simulink model "BaseEngineController_LS_112"  (Simulink 7.7)
settings: Solver=FixedStepDiscrete  StartTime=0.0  StopTime=10.0  RelTol=1e-3
PreLoadFcn:
  | try, eval([bdroot '_setup']); catch, eval('model_setup', ''); end
InitFcn:
  | try, eval([bdroot '_setup']); catch, eval('model_setup', ''); end
undefined symbols (not defined in the file): ECM, H1, H2, High, motohawk_build_version, motohawk_trunc_name, motohawk_vardec_config_group, motohawk_vardec_path, True, xD
libraries: MotoHawk_lib x1417, motohawk_control_primitives_lib x183, motohawk_engine_lib x32, simulink x21, motohawk_annotations_lib x9, AutoDoc_lib x8, simulink_extras x4, motohawk_ccp_examples_lib x1, motohawk_control_primitives_motoshare_lib x1
(part 24 of 27)

== system BaseEngineController_LS_112/Foreground/Control/VirtualSensors/RawProcessed/Base TPS Request/Variable Rate Limiter ==
  note: Rate Limiter - Limit allowable change in signal per timestep
  input : Inport
  rise rate : Inport  Port=2
  fall rate : Inport  Port=3
  Product : Product  SaturateOnIntegerOverflow=on  InputSameDT=on  OutDataTypeStr=Inherit: Same as first input
  Product1 : Product  Inputs=/*  SaturateOnIntegerOverflow=on  InputSameDT=on  OutDataTypeStr=Inherit: Same as first input
  Saturation : motohawk_control_primitives_lib/Saturation  SystemSampleTime=-1
  Sum2 : Sum  Inputs=|++  SaturateOnIntegerOverflow=on  InputSameDT=on  OutDataTypeStr=Inherit: Same as first input
  Sum3 : Sum  Inputs=|+-  SaturateOnIntegerOverflow=on  InputSameDT=on  OutDataTypeStr=Inherit: Same as first input
  Unit Delay : UnitDelay  SampleTime=-1
  motohawk_delta_time : MotoHawk_lib/Extra Development Blocks/motohawk_delta_time  samp_time=-1  init_val=.005  mode=Seconds (double)
  output : Outport  InitialOutput=0
  wires:
  motohawk_delta_time/1 -> Product/1, Product1/1
  Sum3/1 -> Product1/2
  rise rate/1 -> Saturation/3  "Hi Lim"
  fall rate/1 -> Saturation/2  "Lo Lim"
  Product/1 -> Sum2/1
  Sum2/1 -> output/1, Unit Delay/1
  Unit Delay/1 -> Sum2/2, Sum3/2
  Product1/1 -> Saturation/1  "Slope"
  input/1 -> Sum3/1
  Saturation/1 -> Product/2

== system BaseEngineController_LS_112/Foreground/Control/VirtualSensors/RawProcessed/Capture ECT At Startup/Collect Average ==
  note: Collect samples by summing,
      | and divide by the total, to obtain average
  Count : Inport
  Signal : Inport  Port=2
  Enable : EnablePort  StatesWhenEnabling=reset
  Data Type Conversion : DataTypeConversion  SaturateOnIntegerOverflow=on  RndMeth=Zero
  Product : Product  Inputs=/*  OutDataTypeStr=Inherit: Same as first input
  Sum1 : Sum  Inputs=|++  InputSameDT=on
  Unit Delay1 : UnitDelay  SampleTime=-1
  Captured_Signal : Outport
  wires:
  Unit Delay1/1 -> Sum1/2
  Sum1/1 -> Unit Delay1/1, Product/2
  Signal/1 -> Sum1/1
  Product/1 -> Captured_Signal/1
  Count/1 -> Data Type Conversion/1
  Data Type Conversion/1 -> Product/1

== system BaseEngineController_LS_112/Foreground/Control/VirtualSensors/RawProcessed/Capture IAT At Startup/Collect Average ==
  note: Collect samples by summing,
      | and divide by the total, to obtain average
  Count : Inport
  Signal : Inport  Port=2
  Enable : EnablePort  StatesWhenEnabling=reset
  Data Type Conversion : DataTypeConversion  SaturateOnIntegerOverflow=on  RndMeth=Zero
  Product : Product  Inputs=/*  OutDataTypeStr=Inherit: Same as first input
  Sum1 : Sum  Inputs=|++  InputSameDT=on
  Unit Delay1 : UnitDelay  SampleTime=-1
  Captured_Signal : Outport
  wires:
  Data Type Conversion/1 -> Product/1
  Count/1 -> Data Type Conversion/1
  Product/1 -> Captured_Signal/1
  Signal/1 -> Sum1/1
  Sum1/1 -> Product/2, Unit Delay1/1
  Unit Delay1/1 -> Sum1/2

== system BaseEngineController_LS_112/Foreground/Control/VirtualSensors/RawProcessed/EngineState/TDC_Counter ==
  State : Inport
  f : TriggerPort  TriggerType=function-call
  Constant : Constant  OutDataTypeStr=uint8
  Constant1 : Constant  Value=0  OutDataTypeStr=uint8
  Crank State : motohawk_control_primitives_lib/CompareTo  SystemSampleTime=-1  op===  val=2
  CrankCounter : UnitDelay  SampleTime=-1
  Sum : Sum  Inputs=++|  SaturateOnIntegerOverflow=on
  Switch : Switch  Threshold=1  ZeroCross=off  SaturateOnIntegerOverflow=on  InputSameDT=on
  motohawk_probe1 : MotoHawk_lib/Calibration & Probing Blocks/motohawk_probe  nam='CrankTDCs'  show_more=on  name_source=Use Parameter  read_level=1  view_as=Number  enum_struct={'Disabled', 'Enabled'}  vector_style=Wide Row  use_help_units=off  help=''  units=''  use_header_enum=off  row_header_enum={}  col_header_enum={}  use_precision=off  precision=''  gain=1  offset=0  exp=1  use_mototune_group=on  mototune_group=motohawk_vardec_path(gcb)
  CrankCount : Outport
  wires:
  Constant1/1 -> Switch/3
  Sum/1 -> Switch/1
  Switch/1 -> motohawk_probe1/1, CrankCount/1, CrankCounter/1
  Crank State/1 -> Switch/2
  CrankCounter/1 -> Sum/1
  Constant/1 -> Sum/2
  State/1 -> Crank State/1

== system BaseEngineController_LS_112/Foreground/Inputs/LinearSensors/FuelOxygenationSensor/Filter Options/Moving Average Filter ==
  In1 : Inport
  Product{,1..3} (4 alike) : Product  RndMeth=Zero
  Sum : Sum
  Sum1 : Sum  Inputs=++|
  Sum2 : Sum  Inputs=++|
  Unit Delay : UnitDelay  SampleTime=-1
  Unit Delay1 : UnitDelay  SampleTime=-1
  Unit Delay2 : UnitDelay  SampleTime=-1
  motohawk_calibration : MotoHawk_lib/Calibration & Probing Blocks/motohawk_calibration  nam='FinalGain'  val=.5  storage=Calibration  show_more=on  name_source=Use Parameter  data_type=Inherit from 'Default Value'  read_level=1  write_level=1  ovr_cals=on  view_as=Number  enum_struct={'Disabled', 'Enabled'}  vector_style=Wide Row  use_help_units=on  help='Gain 4 For Moving Average Filter'  units=''  use_header_enum=off  row_header_enum={}  col_header_enum={}  use_min_max=off  min_val=-inf  max_val=inf  use_precision=off  precision=''  gain=1  offset=0  exp=1  use_mototune_group=off  mototune_group=motohawk_vardec_path(gcb)
  motohawk_calibration1 : MotoHawk_lib/Calibration & Probing Blocks/motohawk_calibration  nam='Gain1'  val=.5  storage=Calibration  show_more=on  name_source=Use Parameter  data_type=Inherit from 'Default Value'  read_level=1  write_level=1  ovr_cals=on  view_as=Number  enum_struct={'Disabled', 'Enabled'}  vector_style=Wide Row  use_help_units=on  help='Gain 1 For Moving Average Filter'  units=''  use_header_enum=off  row_header_enum={}  col_header_enum={}  use_min_max=off  min_val=-inf  max_val=inf  use_precision=off  precision=''  gain=1  offset=0  exp=1  use_mototune_group=off  mototune_group=motohawk_vardec_path(gcb)
  motohawk_calibration2 : MotoHawk_lib/Calibration & Probing Blocks/motohawk_calibration  nam='Gain2'  val=.3  storage=Calibration  show_more=on  name_source=Use Parameter  data_type=Inherit from 'Default Value'  read_level=1  write_level=1  ovr_cals=on  view_as=Number  enum_struct={'Disabled', 'Enabled'}  vector_style=Wide Row  use_help_units=on  help='Gain 2 For Moving Average Filter'  units=''  use_header_enum=off  row_header_enum={}  col_header_enum={}  use_min_max=off  min_val=-inf  max_val=inf  use_precision=off  precision=''  gain=1  offset=0  exp=1  use_mototune_group=off  mototune_group=motohawk_vardec_path(gcb)
  motohawk_calibration3 : MotoHawk_lib/Calibration & Probing Blocks/motohawk_calibration  nam='Gain3'  val=.2  storage=Calibration  show_more=on  name_source=Use Parameter  data_type=Inherit from 'Default Value'  read_level=1  write_level=1  ovr_cals=on  view_as=Number  enum_struct={'Disabled', 'Enabled'}  vector_style=Wide Row  use_help_units=on  help='Gain 3 For Moving Average Filter'  units=''  use_header_enum=off  row_header_enum={}  col_header_enum={}  use_min_max=off  min_val=-inf  max_val=inf  use_precision=off  precision=''  gain=1  offset=0  exp=1  use_mototune_group=off  mototune_group=motohawk_vardec_path(gcb)
  Out1 : Outport
  wires:
  Sum/1 -> Product/2
  Product/1 -> Out1/1
  motohawk_calibration/1 -> Product/1
  In1/1 -> Sum/1, Unit Delay/1
  Unit Delay/1 -> Unit Delay1/1, Product1/2
  Unit Delay1/1 -> Unit Delay2/1, Product2/2
  Unit Delay2/1 -> Product3/2
  motohawk_calibration1/1 -> Product1/1
  motohawk_calibration3/1 -> Product3/1
  motohawk_calibration2/1 -> Product2/1
  Product1/1 -> Sum1/1
  Product2/1 -> Sum2/1
  Sum2/1 -> Sum1/2
  Sum1/1 -> Sum/2
  Product3/1 -> Sum2/2

== system BaseEngineController_LS_112/Foreground/Inputs/LinearSensors/FuelOxygenationSensor/Filter Options/Rate Limiter ==
  In1 : Inport
  Variable Rate Limiter : motohawk_control_primitives_motoshare_lib/Variable Rate Limiter  SystemSampleTime=-1
  motohawk_calibration : MotoHawk_lib/Calibration & Probing Blocks/motohawk_calibration  nam='Rise_Rate'  val=.025  storage=Calibration  show_more=off  name_source=Use Parameter  data_type=Inherit from 'Default Value'  read_level=1  write_level=1  ovr_cals=on  view_as=Number  enum_struct={'Disabled', 'Enabled'}  vector_style=Wide Row  use_help_units=off  help=''  units=''  use_header_enum=off  row_header_enum={}  col_header_enum={}  use_min_max=off  min_val=-inf  max_val=inf  use_precision=off  precision=''  gain=1  offset=0  exp=1  use_mototune_group=off  mototune_group=motohawk_vardec_path(gcb)
  motohawk_calibration1 : MotoHawk_lib/Calibration & Probing Blocks/motohawk_calibration  nam='Fall_Rate'  val=.025  storage=Calibration  show_more=off  name_source=Use Parameter  data_type=Inherit from 'Default Value'  read_level=1  write_level=1  ovr_cals=on  view_as=Number  enum_struct={'Disabled', 'Enabled'}  vector_style=Wide Row  use_help_units=off  help=''  units=''  use_header_enum=off  row_header_enum={}  col_header_enum={}  use_min_max=off  min_val=-inf  max_val=inf  use_precision=off  precision=''  gain=1  offset=0  exp=1  use_mototune_group=off  mototune_group=motohawk_vardec_path(gcb)
  Out1 : Outport
  wires:
  Variable Rate Limiter/1 -> Out1/1
  In1/1 -> Variable Rate Limiter/1
  motohawk_calibration/1 -> Variable Rate Limiter/2
  motohawk_calibration1/1 -> Variable Rate Limiter/3

== system BaseEngineController_LS_112/Foreground/Outputs/AEM Infinity Dash/Dash Message 2/PHI_Filt/DecreasingFilter ==
  Enable : EnablePort
  motohawk_calibration2 : MotoHawk_lib/Calibration & Probing Blocks/motohawk_calibration  nam='PH1_FiltDecConst'  val=1.25  storage=Calibration  show_more=on  name_source=Use Parameter  data_type=Inherit from 'Default Value'  read_level=1  write_level=1  ovr_cals=on  view_as=Number  enum_struct={'Disabled', 'Enabled'}  vector_style=Wide Row  use_help_units=on  help='Filter time constant for a decreasing signal.'  units='sec'  use_header_enum=off  row_header_enum={}  col_header_enum={}  use_min_max=off  min_val=-inf  max_val=inf  use_precision=off  precision=''  gain=1  offset=0  exp=1  use_mototune_group=on  mototune_group=motohawk_vardec_path(gcb)
  Out1 : Outport  InitialOutput=.005
  wires:
  motohawk_calibration2/1 -> Out1/1

== system BaseEngineController_LS_112/Foreground/Outputs/AEM Infinity Dash/Dash Message 2/PHI_Filt/IncreasingFilter ==
  Enable : EnablePort
  motohawk_calibration1 : MotoHawk_lib/Calibration & Probing Blocks/motohawk_calibration  nam='PH1_FiltIncConst'  val=1.25  storage=Calibration  show_more=on  name_source=Use Parameter  data_type=Inherit from 'Default Value'  read_level=1  write_level=1  ovr_cals=on  view_as=Number  enum_struct={'Disabled', 'Enabled'}  vector_style=Wide Row  use_help_units=on  help='Filter time constant for a increasing signal.'  units='sec'  use_header_enum=off  row_header_enum={}  col_header_enum={}  use_min_max=off  min_val=-inf  max_val=inf  use_precision=off  precision=''  gain=1  offset=0  exp=1  use_mototune_group=on  mototune_group=motohawk_vardec_path(gcb)
  Out1 : Outport  InitialOutput=.005
  wires:
  motohawk_calibration1/1 -> Out1/1

== system BaseEngineController_LS_112/Foreground/Outputs/AEM Infinity Dash/Dash Message 2/PHI_Filt1/DecreasingFilter ==
  Enable : EnablePort
  motohawk_calibration2 : MotoHawk_lib/Calibration & Probing Blocks/motohawk_calibration  nam='PH2_FiltDecConst'  val=1.25  storage=Calibration  show_more=on  name_source=Use Parameter  data_type=Inherit from 'Default Value'  read_level=1  write_level=1  ovr_cals=on  view_as=Number  enum_struct={'Disabled', 'Enabled'}  vector_style=Wide Row  use_help_units=on  help='Filter time constant for a decreasing signal.'  units='sec'  use_header_enum=off  row_header_enum={}  col_header_enum={}  use_min_max=off  min_val=-inf  max_val=inf  use_precision=off  precision=''  gain=1  offset=0  exp=1  use_mototune_group=on  mototune_group=motohawk_vardec_path(gcb)
  Out1 : Outport  InitialOutput=.005
  wires:
  motohawk_calibration2/1 -> Out1/1

== system BaseEngineController_LS_112/Foreground/Outputs/AEM Infinity Dash/Dash Message 2/PHI_Filt1/IncreasingFilter ==
  Enable : EnablePort
  motohawk_calibration1 : MotoHawk_lib/Calibration & Probing Blocks/motohawk_calibration  nam='PH2_FiltIncConst'  val=1.25  storage=Calibration  show_more=on  name_source=Use Parameter  data_type=Inherit from 'Default Value'  read_level=1  write_level=1  ovr_cals=on  view_as=Number  enum_struct={'Disabled', 'Enabled'}  vector_style=Wide Row  use_help_units=on  help='Filter time constant for a increasing signal.'  units='sec'  use_header_enum=off  row_header_enum={}  col_header_enum={}  use_min_max=off  min_val=-inf  max_val=inf  use_precision=off  precision=''  gain=1  offset=0  exp=1  use_mototune_group=on  mototune_group=motohawk_vardec_path(gcb)
  Out1 : Outport  InitialOutput=.005
  wires:
  motohawk_calibration1/1 -> Out1/1

== system BaseEngineController_LS_112/Foreground/Outputs/Coil Control/Coil Enable Manager/EST Enable TDC Counter/TDC_Counter ==
  Reset : Inport
  f : TriggerPort  TriggerType=function-call
  Constant : Constant  OutDataTypeStr=uint8
  Constant1 : Constant  Value=0  OutDataTypeStr=uint8
  CrankCounter : UnitDelay  SampleTime=-1
  Sum : Sum  Inputs=|++  SaturateOnIntegerOverflow=on
  Switch1 : Switch  Threshold=1  ZeroCross=off  SaturateOnIntegerOverflow=on  InputSameDT=on
  CrankCount : Outport
  wires:
  Constant1/1 -> Switch1/1
  Sum/1 -> Switch1/3
  Reset/1 -> Switch1/2
  Switch1/1 -> CrankCount/1, CrankCounter/1
  Constant/1 -> Sum/1
  CrankCounter/1 -> Sum/2

== system BaseEngineController_LS_112/Foreground/Control/ActuatorCharacterization/Electronic Throttle Controller/PID With Damper Terms (Tunable)/DamperSwitch/Filtered Derivative ==
  Raw : Inport
  Derivitive2 : motohawk_control_primitives_lib/Derivitive  SystemSampleTime=-1  samp_time=.005
  First Order Low Pass (Tunable) : motohawk_control_primitives_lib/First Order Low Pass (Tunable)  SystemSampleTime=-1  nam=[prefix 'DamperTPSFilt']  samp_time=-1  group=[grp ' | ' prefix ' PID Config']
  Filt_Deriv : Outport
  wires:
  Raw/1 -> First Order Low Pass (Tunable)/1
  Derivitive2/1 -> Filt_Deriv/1
  First Order Low Pass (Tunable)/1 -> Derivitive2/1

== system BaseEngineController_LS_112/Foreground/Control/Controller/Run/AC Control/AC Comp High Pressure/Hysteresis ==
  note: Hi & !Lo => Hi
      | Lo & !Hi => Lo
      | Otherwise, Hold
  Hi : Inport
  Lo : Inport  Port=2
  Combinatorial  Logic : CombinatorialLogic  TruthTable=[0 0;0 1;1 1;0 0]
  Demux : Demux  Outputs=2
  Mux : Mux  Inputs=2
  Switch1 : Switch  Threshold=0.5  SaturateOnIntegerOverflow=on  InputSameDT=on
  Unit Delay : UnitDelay  SampleTime=-1
  "Out (Lo=0, Hi=1)" : Outport
  wires:
  Mux/1 -> Combinatorial  Logic/1
  Combinatorial  Logic/1 -> Demux/1
  Demux/1 -> Switch1/1
  Demux/2 -> Switch1/2
  Unit Delay/1 -> Switch1/3
  Switch1/1 -> Unit Delay/1, "Out (Lo=0, Hi=1)"/1
  Hi/1 -> Mux/1
  Lo/1 -> Mux/2

== system BaseEngineController_LS_112/Foreground/Control/Controller/Run/AC Control/AC Comp Low Pressure/Hysteresis ==
  note: Hi & !Lo => Hi
      | Lo & !Hi => Lo
      | Otherwise, Hold
  Hi : Inport
  Lo : Inport  Port=2
  Combinatorial  Logic : CombinatorialLogic  TruthTable=[0 0;0 1;1 1;0 0]
  Demux : Demux  Outputs=2
  Mux : Mux  Inputs=2
  Switch1 : Switch  Threshold=0.5  SaturateOnIntegerOverflow=on  InputSameDT=on
  Unit Delay : UnitDelay  SampleTime=-1
  "Out (Lo=0, Hi=1)" : Outport
  wires:
  Mux/1 -> Combinatorial  Logic/1
  Combinatorial  Logic/1 -> Demux/1
  Demux/1 -> Switch1/1
  Demux/2 -> Switch1/2
  Unit Delay/1 -> Switch1/3
  Switch1/1 -> Unit Delay/1, "Out (Lo=0, Hi=1)"/1
  Hi/1 -> Mux/1
  Lo/1 -> Mux/2

== system BaseEngineController_LS_112/Foreground/Control/Controller/Run/AC Control/AC Comp Overspeed/Hysteresis ==
  note: Hi & !Lo => Hi
      | Lo & !Hi => Lo
      | Otherwise, Hold
  Hi : Inport
  Lo : Inport  Port=2
  Combinatorial  Logic : CombinatorialLogic  TruthTable=[0 0;0 1;1 1;0 0]
  Demux : Demux  Outputs=2
  Mux : Mux  Inputs=2
  Switch1 : Switch  Threshold=0.5  SaturateOnIntegerOverflow=on  InputSameDT=on
  Unit Delay : UnitDelay  SampleTime=-1
  "Out (Lo=0, Hi=1)" : Outport
  wires:
  Mux/1 -> Combinatorial  Logic/1
  Combinatorial  Logic/1 -> Demux/1
  Demux/1 -> Switch1/1
  Demux/2 -> Switch1/2
  Unit Delay/1 -> Switch1/3
  Switch1/1 -> Unit Delay/1, "Out (Lo=0, Hi=1)"/1
  Hi/1 -> Mux/1
  Lo/1 -> Mux/2

== system BaseEngineController_LS_112/Foreground/Control/Controller/Run/AC Control/AC Comp Overspeed1/Hysteresis ==
  note: Hi & !Lo => Hi
      | Lo & !Hi => Lo
      | Otherwise, Hold
  Hi : Inport
  Lo : Inport  Port=2
  Combinatorial  Logic : CombinatorialLogic  TruthTable=[0 0;0 1;1 1;0 0]
  Demux : Demux  Outputs=2
  Mux : Mux  Inputs=2
  Switch1 : Switch  Threshold=0.5  SaturateOnIntegerOverflow=on  InputSameDT=on
  Unit Delay : UnitDelay  SampleTime=-1
  "Out (Lo=0, Hi=1)" : Outport
  wires:
  Mux/1 -> Combinatorial  Logic/1
  Combinatorial  Logic/1 -> Demux/1
  Demux/1 -> Switch1/1
  Demux/2 -> Switch1/2
  Unit Delay/1 -> Switch1/3
  Switch1/1 -> Unit Delay/1, "Out (Lo=0, Hi=1)"/1
  Hi/1 -> Mux/1
  Lo/1 -> Mux/2

== system BaseEngineController_LS_112/Foreground/Control/Controller/Run/AC Control/AC Comp Underspeed/Hysteresis ==
  note: Hi & !Lo => Hi
      | Lo & !Hi => Lo
      | Otherwise, Hold
  Hi : Inport
  Lo : Inport  Port=2
  Combinatorial  Logic : CombinatorialLogic  TruthTable=[0 0;0 1;1 1;0 0]
  Demux : Demux  Outputs=2
  Mux : Mux  Inputs=2
  Switch1 : Switch  Threshold=0.5  SaturateOnIntegerOverflow=on  InputSameDT=on
  Unit Delay : UnitDelay  SampleTime=-1
  "Out (Lo=0, Hi=1)" : Outport
  wires:
  Mux/1 -> Combinatorial  Logic/1
  Combinatorial  Logic/1 -> Demux/1
  Demux/1 -> Switch1/1
  Demux/2 -> Switch1/2
  Unit Delay/1 -> Switch1/3
  Switch1/1 -> Unit Delay/1, "Out (Lo=0, Hi=1)"/1
  Hi/1 -> Mux/1
  Lo/1 -> Mux/2

== system BaseEngineController_LS_112/Foreground/Control/Controller/Run/AC Control/AC Evap Temp Hyst/Hysteresis ==
  note: Hi & !Lo => Hi
      | Lo & !Hi => Lo
      | Otherwise, Hold
  Hi : Inport
  Lo : Inport  Port=2
  Combinatorial  Logic : CombinatorialLogic  TruthTable=[0 0;0 1;1 1;0 0]
  Demux : Demux  Outputs=2
  Mux : Mux  Inputs=2
  Switch1 : Switch  Threshold=0.5  SaturateOnIntegerOverflow=on  InputSameDT=on
  Unit Delay : UnitDelay  SampleTime=-1
  "Out (Lo=0, Hi=1)" : Outport
  wires:
  Mux/1 -> Combinatorial  Logic/1
  Combinatorial  Logic/1 -> Demux/1
  Demux/1 -> Switch1/1
  Demux/2 -> Switch1/2
  Unit Delay/1 -> Switch1/3
  Switch1/1 -> Unit Delay/1, "Out (Lo=0, Hi=1)"/1
  Hi/1 -> Mux/1
  Lo/1 -> Mux/2

== system BaseEngineController_LS_112/Foreground/Control/Controller/Run/Boost Control/BoostControl Adapt/Adapt Boost Table ==
  error : Inport
  Enable : EnablePort
  Documentation_Calibrations_Probes_Block : AutoDoc_lib/Documentation_Calibrations_Probes_Block
  Documentation_Left_Border : AutoDoc_lib/Documentation_Left_Border  layout=Portrait
  Documentation_Right_Border : AutoDoc_lib/Documentation_Right_Border  layout=Portrait
  motohawk_adapt_table : MotoHawk_lib/Lookup Tables/motohawk_adapt_table  nam='BoostControlBase_AdaptMap'  typ=double  mode=Adapt between points  show_adapted=off
  motohawk_calibration1 : MotoHawk_lib/Calibration & Probing Blocks/motohawk_calibration  nam='BoostControlOfstMinValue'  val=0  storage=Calibration  show_more=on  name_source=Use Parameter  data_type=double  read_level=1  write_level=1  ovr_cals=on  view_as=Number  enum_struct={'Disabled', 'Enabled'}  vector_style=Wide Row  use_help_units=on  help='Minimum value that can be adapted into the BaseAirflowOfst table.'  units='%'  use_header_enum=off  row_header_enum={}  col_header_enum={}  use_min_max=on  min_val=-inf  max_val=inf  use_precision=off  precision=''  gain=1  offset=0  exp=1  use_mototune_group=on  mototune_group=motohawk_vardec_path(gcb)
  motohawk_calibration2 : MotoHawk_lib/Calibration & Probing Blocks/motohawk_calibration  nam='BoostControlOfstMaxValue'  val=0  storage=Calibration  show_more=on  name_source=Use Parameter  data_type=double  read_level=1  write_level=1  ovr_cals=on  view_as=Number  enum_struct={'Disabled', 'Enabled'}  vector_style=Wide Row  use_help_units=on  help='Maximum value that can be adapted into the BaseAirflowOfst table.'  units='%'  use_header_enum=off  row_header_enum={}  col_header_enum={}  use_min_max=on  min_val=-inf  max_val=inf  use_precision=off  precision=''  gain=1  offset=0  exp=1  use_mototune_group=on  mototune_group=motohawk_vardec_path(gcb)
  wires:
  error/1 -> motohawk_adapt_table/1
  motohawk_calibration1/1 -> motohawk_adapt_table/2
  motohawk_calibration2/1 -> motohawk_adapt_table/3

== system BaseEngineController_LS_112/Foreground/Control/Controller/Run/Boost Control/BoostControl Adapt/BoostControl Enable Delay ==
  State_In : Inport
  Relational Operator : RelationalOperator  Operator=>  InputSameDT=on
  Time Since Enabled (With Input)1 : motohawk_control_primitives_lib/Time Since Enabled (With Input)1  SystemSampleTime=-1  nam='BoostTimer'  samp_time=.005  init=0  upperlim=16000
  motohawk_calibration1 : MotoHawk_lib/Calibration & Probing Blocks/motohawk_calibration  nam='BoostAdaptDelayTime'  val=5  storage=Calibration  show_more=on  name_source=Use Parameter  data_type=Inherit from 'Default Value'  read_level=1  write_level=1  ovr_cals=on  view_as=Number  enum_struct={'Disabled', 'Enabled'}  vector_style=Wide Row  use_help_units=on  help='Idle Control must be enabled for this amount of time before fuel adaption is enabled'  units='s'  use_header_enum=off  row_header_enum={}  col_header_enum={}  use_min_max=off  min_val=0  max_val=inf  use_precision=off  precision=''  gain=1  offset=0  exp=1  use_mototune_group=on  mototune_group=motohawk_vardec_path(gcb)
  State_Out : Outport
  wires:
  State_In/1 -> Time Since Enabled (With Input)1/1
  motohawk_calibration1/1 -> Relational Operator/2
  Time Since Enabled (With Input)1/1 -> Relational Operator/1
  Relational Operator/1 -> State_Out/1

== system BaseEngineController_LS_112/Foreground/Control/Controller/Run/Boost Control/BoostControl Adapt/Saturation (Tunable) ==
  note: Calibratable wrapper around the Saturation block
  In : Inport
  Saturation : motohawk_control_primitives_lib/Saturation  SystemSampleTime=-1
  motohawk_calibration : MotoHawk_lib/Calibration & Probing Blocks/motohawk_calibration  nam=[prefix 'LwrLim']  val=LwrLim  storage=Calibration  show_more=on  name_source=Use Parameter  data_type=Inherit via back propagation  read_level=1  write_level=1  ovr_cals=on  view_as=Number  enum_struct={'Disabled', 'Enabled'}  vector_style=Wide Row  use_help_units=off  help='Lower Limit Value'  units=units  use_header_enum=off  row_header_enum={}  col_header_enum={}  use_min_max=on  min_val=-inf  max_val=inf  use_precision=on  precision='1.4'  gain=1  offset=0  exp=1  use_mototune_group=on  mototune_group=motohawk_vardec_path(gcb)
  motohawk_calibration1 : MotoHawk_lib/Calibration & Probing Blocks/motohawk_calibration  nam=[prefix 'UprLim']  val=UprLim  storage=Calibration  show_more=on  name_source=Use Parameter  data_type=Inherit via back propagation  read_level=1  write_level=1  ovr_cals=on  view_as=Number  enum_struct={'Disabled', 'Enabled'}  vector_style=Wide Row  use_help_units=off  help='Upper Limit Value'  units=units  use_header_enum=off  row_header_enum={}  col_header_enum={}  use_min_max=on  min_val=-inf  max_val=inf  use_precision=on  precision='1.4'  gain=1  offset=0  exp=1  use_mototune_group=on  mototune_group=motohawk_vardec_path(gcb)
  Out : Outport
  wires:
  motohawk_calibration1/1 -> Saturation/3
  In/1 -> Saturation/1
  motohawk_calibration/1 -> Saturation/2
  Saturation/1 -> Out/1

== system BaseEngineController_LS_112/Foreground/Control/Controller/Run/Boost Control/Universal PID (Tunable & Scheduled)/PID Gain Select1 ==
  ErrorIdx : Inport
  Product1 : Product  SaturateOnIntegerOverflow=on  InputSameDT=on  OutDataTypeStr=Inherit: Same as first input
  Product2 : Product  SaturateOnIntegerOverflow=on  InputSameDT=on  OutDataTypeStr=Inherit: Same as first input
  Product3 : Product  SaturateOnIntegerOverflow=on  InputSameDT=on  OutDataTypeStr=Inherit: Same as first input
  motohawk_calibration1 : MotoHawk_lib/Calibration & Probing Blocks/motohawk_calibration  nam=[prefix 'IGain']  val=0  storage=Calibration  show_more=on  name_source=Use Parameter  data_type=Inherit from 'Default Value'  read_level=1  write_level=1  ovr_cals=on  view_as=Number  enum_struct={'Disabled', 'Enabled'}  vector_style=Wide Row  use_help_units=on  help='Base I-gain for the min. governor controller.'  units='mult'  use_header_enum=off  row_header_enum={}  col_header_enum={}  use_min_max=off  min_val=-inf  max_val=inf  use_precision=off  precision=''  gain=1  offset=0  exp=1  use_mototune_group=on  mototune_group=motohawk_vardec_path(gcb)
  motohawk_calibration2 : MotoHawk_lib/Calibration & Probing Blocks/motohawk_calibration  nam=[prefix 'DGain']  val=0  storage=Calibration  show_more=on  name_source=Use Parameter  data_type=Inherit from 'Default Value'  read_level=1  write_level=1  ovr_cals=on  view_as=Number  enum_struct={'Disabled', 'Enabled'}  vector_style=Wide Row  use_help_units=on  help='Base D-gain for the min. governor controller.'  units='mult'  use_header_enum=off  row_header_enum={}  col_header_enum={}  use_min_max=off  min_val=-inf  max_val=inf  use_precision=off  precision=''  gain=1  offset=0  exp=1  use_mototune_group=on  mototune_group=motohawk_vardec_path(gcb)
  motohawk_calibration3 : MotoHawk_lib/Calibration & Probing Blocks/motohawk_calibration  nam=[prefix 'PGain']  val=0  storage=Calibration  show_more=on  name_source=Use Parameter  data_type=Inherit from 'Default Value'  read_level=1  write_level=1  ovr_cals=on  view_as=Number  enum_struct={'Disabled', 'Enabled'}  vector_style=Wide Row  use_help_units=on  help='Base P-gain for the min. governor controller.'  units='mult'  use_header_enum=off  row_header_enum={}  col_header_enum={}  use_min_max=off  min_val=-inf  max_val=inf  use_precision=off  precision=''  gain=1  offset=0  exp=1  use_mototune_group=on  mototune_group=motohawk_vardec_path(gcb)
  motohawk_interpolation_1d1 : MotoHawk_lib/Lookup Tables/motohawk_interpolation_1d  nam=[prefix 'IGainErrorMult']  table_data=[0.5 0.3 0.01 0.01 0.2 0.5 1 1.3 1.5]  show_more=on  data_type=Inherit from 'Table Data'  storage=NonAdaptive  read_level=1  write_level=1  ovr_cals=on  use_help=on  help=''  units='mult'  use_min_max=on  min_val=-inf  max_val=inf  use_precision=off  precision=''  gain=1  offset=0  exp=1  use_links=off  prelookup_block=''  output_name=''  use_mototune_group=on  mototune_group=motohawk_vardec_path(gcb)
  motohawk_interpolation_1d2 : MotoHawk_lib/Lookup Tables/motohawk_interpolation_1d  nam=[prefix 'PGainErrorMult']  table_data=[0.5 0.3 0.01 0.01 0.2 0.5 1 1.3 1.5]  show_more=on  data_type=Inherit from 'Table Data'  storage=NonAdaptive  read_level=1  write_level=1  ovr_cals=on  use_help=on  help=''  units='mult'  use_min_max=on  min_val=-inf  max_val=inf  use_precision=off  precision=''  gain=1  offset=0  exp=1  use_links=off  prelookup_block=''  output_name=''  use_mototune_group=on  mototune_group=motohawk_vardec_path(gcb)
  motohawk_interpolation_1d3 : MotoHawk_lib/Lookup Tables/motohawk_interpolation_1d  nam=[prefix 'DGainErrorMult']  table_data=[0.5 0.3 0.01 0.01 0.2 0.5 1 1.3 1.5]  show_more=on  data_type=Inherit from 'Table Data'  storage=NonAdaptive  read_level=1  write_level=1  ovr_cals=on  use_help=on  help=''  units='mult'  use_min_max=on  min_val=-inf  max_val=inf  use_precision=off  precision=''  gain=1  offset=0  exp=1  use_links=off  prelookup_block=''  output_name=''  use_mototune_group=on  mototune_group=motohawk_vardec_path(gcb)
  PGain : Outport
  IGain : Outport  Port=2
  DGain : Outport  Port=3
  wires:
  ErrorIdx/1 -> motohawk_interpolation_1d2/1, motohawk_interpolation_1d1/1, motohawk_interpolation_1d3/1
  motohawk_interpolation_1d2/1 -> Product2/2
  Product2/1 -> PGain/1
  motohawk_calibration3/1 -> Product2/1
  motohawk_calibration1/1 -> Product1/1
  motohawk_interpolation_1d1/1 -> Product1/2
  Product1/1 -> IGain/1
  motohawk_interpolation_1d3/1 -> Product3/2
  Product3/1 -> DGain/1
  motohawk_calibration2/1 -> Product3/1

== system BaseEngineController_LS_112/Foreground/Control/Controller/Run/FAN Control/Hysterisis/Hysteresis ==
  note: Hi & !Lo => Hi
      | Lo & !Hi => Lo
      | Otherwise, Hold
  Hi : Inport
  Lo : Inport  Port=2
  Combinatorial  Logic : CombinatorialLogic  TruthTable=[0 0;0 1;1 1;0 0]
  Demux : Demux  Outputs=2
  Mux : Mux  Inputs=2
  Switch1 : Switch  Threshold=0.5  SaturateOnIntegerOverflow=on  InputSameDT=on
  Unit Delay : UnitDelay  SampleTime=-1
  "Out (Lo=0, Hi=1)" : Outport
  wires:
  Mux/1 -> Combinatorial  Logic/1
  Combinatorial  Logic/1 -> Demux/1
  Demux/1 -> Switch1/1
  Demux/2 -> Switch1/2
  Unit Delay/1 -> Switch1/3
  Switch1/1 -> Unit Delay/1, "Out (Lo=0, Hi=1)"/1
  Hi/1 -> Mux/1
  Lo/1 -> Mux/2

== system BaseEngineController_LS_112/Foreground/Control/Controller/Run/FAN Control/Hysterisis1/Hysteresis ==
  note: Hi & !Lo => Hi
      | Lo & !Hi => Lo
      | Otherwise, Hold
  Hi : Inport
  Lo : Inport  Port=2
  Combinatorial  Logic : CombinatorialLogic  TruthTable=[0 0;0 1;1 1;0 0]
  Demux : Demux  Outputs=2
  Mux : Mux  Inputs=2
  Switch1 : Switch  Threshold=0.5  SaturateOnIntegerOverflow=on  InputSameDT=on
  Unit Delay : UnitDelay  SampleTime=-1
  "Out (Lo=0, Hi=1)" : Outport
  wires:
  Mux/1 -> Combinatorial  Logic/1
  Combinatorial  Logic/1 -> Demux/1
  Demux/1 -> Switch1/1
  Demux/2 -> Switch1/2
  Unit Delay/1 -> Switch1/3
  Switch1/1 -> Unit Delay/1, "Out (Lo=0, Hi=1)"/1
  Hi/1 -> Mux/1
  Lo/1 -> Mux/2

== system BaseEngineController_LS_112/Foreground/Control/Controller/Run/FAN Control/Hysterisis2/Hysteresis ==
  note: Hi & !Lo => Hi
      | Lo & !Hi => Lo
      | Otherwise, Hold
  Hi : Inport
  Lo : Inport  Port=2
  Combinatorial  Logic : CombinatorialLogic  TruthTable=[0 0;0 1;1 1;0 0]
  Demux : Demux  Outputs=2
  Mux : Mux  Inputs=2
  Switch1 : Switch  Threshold=0.5  SaturateOnIntegerOverflow=on  InputSameDT=on
  Unit Delay : UnitDelay  SampleTime=-1
  "Out (Lo=0, Hi=1)" : Outport
  wires:
  Mux/1 -> Combinatorial  Logic/1
  Combinatorial  Logic/1 -> Demux/1
  Demux/1 -> Switch1/1
  Demux/2 -> Switch1/2
  Unit Delay/1 -> Switch1/3
  Switch1/1 -> Unit Delay/1, "Out (Lo=0, Hi=1)"/1
  Hi/1 -> Mux/1
  Lo/1 -> Mux/2

== system BaseEngineController_LS_112/Foreground/Control/Controller/Run/Fuel System Manager/Fuel Calculation/Calculate Fuel Flow ==
  DesEquivRatio : Inport
  Sensors : Inport  Port=2
  Bus Selector1 : BusSelector  OutputSignals=AirCalcs.MAFPort,Raw.LinearSensors.FuelSense
  Calculate A/F Ratio : Subsystem
  Fuel Flow = Mass Airflow * Equivalence Ratio / Air-to-fuel Ratio : Product  Inputs=**/  SaturateOnIntegerOverflow=on  InputSameDT=on  OutDataTypeStr=Inherit: Same as first input
  Gasoline Stoich A/F Ratio : Constant  Value=14.6
  Terminator9 : Terminator
  motohawk_probe1 : MotoHawk_lib/Calibration & Probing Blocks/motohawk_probe  nam='Desired_AF_Ratio'  show_more=on  name_source=Use Parameter  read_level=1  view_as=Number  enum_struct={'Disabled', 'Enabled'}  vector_style=Wide Row  use_help_units=on  help='Desired Air to Fuel Ratio based on Ethanol Percentage'  units='ratio'  use_header_enum=off  row_header_enum={}  col_header_enum={}  use_precision=on  precision='5.2'  gain=1  offset=0  exp=1  use_mototune_group=on  mototune_group=motohawk_vardec_path(gcb)
  BaseFuelRate [g/s] : Outport
  wires:
  DesEquivRatio/1 -> Fuel Flow = Mass Airflow * Equivalence Ratio / Air-to-fuel Ratio/2
  Sensors/1 -> Bus Selector1/1
  Bus Selector1/1 -> Fuel Flow = Mass Airflow * Equivalence Ratio / Air-to-fuel Ratio/1  "<MAFPort>"
  Fuel Flow = Mass Airflow * Equivalence Ratio / Air-to-fuel Ratio/1 -> BaseFuelRate [g/s]/1
  Calculate A/F Ratio/1(Desired A/F Ratio) -> Fuel Flow = Mass Airflow * Equivalence Ratio / Air-to-fuel Ratio/3, motohawk_probe1/1
  Bus Selector1/2 -> Calculate A/F Ratio/1(Ethanol_xx [%])  "<FuelSense>"
  Gasoline Stoich A/F Ratio/1 -> Terminator9/1

== system BaseEngineController_LS_112/Foreground/Control/Controller/Run/Fuel System Manager/Injector Manager/Delta TPS Transient Fueling ==
  TPS : Inport
  MAF : Inport  Port=2
  ECTIdx : Inport  Port=3
  MAPAngle : Inport  Port=4
  OxyIdx : Inport  Port=5
  Enable : EnablePort  StatesWhenEnabling=reset
  CompareTo1 : motohawk_control_primitives_lib/CompareTo  SystemSampleTime=-1  op=~=  val=1
  CompareTo2 : motohawk_control_primitives_lib/CompareTo  SystemSampleTime=-1  op=~=  val=1
  ECT Transient Fueling : Subsystem  TreatAsAtomicUnit=on
  First Order Low Pass (Tunable) : motohawk_control_primitives_lib/First Order Low Pass (Tunable)  SystemSampleTime=-1  nam='DeltaTPS_FiltConst'  samp_time=-1  group=motohawk_vardec_path(gcb)
  First Order Low Pass (Tunable)1 : motohawk_control_primitives_lib/First Order Low Pass (Tunable)  SystemSampleTime=-1  nam='DeltaMAP_FiltConst'  samp_time=-1  group=motohawk_vardec_path(gcb)
  Logical Operator : Logic  Operator=OR  AllPortsSameDT=off  OutDataTypeStr=boolean
  OXY Transient Fueling : Subsystem  TreatAsAtomicUnit=on
  Product1 : Product  Inputs=4  SaturateOnIntegerOverflow=on  OutDataTypeStr=Inherit: Same as first input
  Sum : Sum  Inputs=|+-  SaturateOnIntegerOverflow=on
  Sum1 : Sum  Inputs=|+-  SaturateOnIntegerOverflow=on
  motohawk_interpolation_2d1 : MotoHawk_lib/Lookup Tables/motohawk_interpolation_2d  nam='DeltaMAP_Mult'  table_data=ones(9,17)  show_more=on  data_type=Inherit from 'Table Data'  storage=NonAdaptive  read_level=1  write_level=1  ovr_cals=on  use_help=on  help='Transient Fueling Multiplier for adjustment based on delta MAP'  units='mult'  use_min_max=off  min_val=-inf  max_val=inf  use_precision=on  precision=''  gain=1  offset=0  exp=1  use_links=off  row_prelookup_block=''  col_prelookup_block=''  output_name=''  use_mototune_group=on  mototune_group=motohawk_vardec_path(gcb)
  motohawk_interpolation_2d2 : MotoHawk_lib/Lookup Tables/motohawk_interpolation_2d  nam='DeltaTPS_Mult'  table_data=ones(9,17)  show_more=on  data_type=Inherit from 'Table Data'  storage=NonAdaptive  read_level=1  write_level=1  ovr_cals=on  use_help=on  help='Transient Fueling Multiplier for adjustment based on delta TPS'  units='mult'  use_min_max=off  min_val=-inf  max_val=inf  use_precision=on  precision=''  gain=1  offset=0  exp=1  use_links=off  row_prelookup_block=''  col_prelookup_block=''  output_name=''  use_mototune_group=on  mototune_group=motohawk_vardec_path(gcb)
  motohawk_prelookup : MotoHawk_lib/Lookup Tables/motohawk_prelookup  nam='MAF09'  breakpoint_data=ones(1,9)  show_more=on  data_type=Inherit from 'Table Data'  storage=Constant  read_level=1  write_level=1  ovr_cals=on  use_help=off  help=''  units=''  use_min_max=off  min_val=-inf  max_val=inf  use_precision=off  precision=''  gain=1  offset=0  exp=1  use_links=off  input_name=''  use_mototune_group=on  mototune_group=motohawk_vardec_path(gcb)
  motohawk_prelookup1 : MotoHawk_lib/Lookup Tables/motohawk_prelookup  nam='DeltaTPS17'  breakpoint_data=ones(1,17)  show_more=on  data_type=Inherit from 'Table Data'  storage=Constant  read_level=1  write_level=1  ovr_cals=on  use_help=off  help=''  units=''  use_min_max=off  min_val=-inf  max_val=inf  use_precision=off  precision=''  gain=1  offset=0  exp=1  use_links=off  input_name=''  use_mototune_group=on  mototune_group=motohawk_vardec_path(gcb)
  motohawk_prelookup3 : MotoHawk_lib/Lookup Tables/motohawk_prelookup  nam='DeltaMAP17'  breakpoint_data=ones(1,17)  show_more=on  data_type=Inherit from 'Table Data'  storage=Constant  read_level=1  write_level=1  ovr_cals=on  use_help=off  help=''  units=''  use_min_max=off  min_val=-inf  max_val=inf  use_precision=off  precision=''  gain=1  offset=0  exp=1  use_links=off  input_name=''  use_mototune_group=on  mototune_group=motohawk_vardec_path(gcb)
  motohawk_probe1 : MotoHawk_lib/Calibration & Probing Blocks/motohawk_probe  nam='DeltaMAP'  show_more=on  name_source=Use Parameter  read_level=1  view_as=Number  enum_struct={'Disabled', 'Enabled'}  vector_style=Wide Row  use_help_units=off  help=''  units=''  use_header_enum=off  row_header_enum={}  col_header_enum={}  use_precision=off  precision=''  gain=1  offset=0  exp=1  use_mototune_group=on  mototune_group=motohawk_vardec_path(gcb)
  motohawk_probe2 : MotoHawk_lib/Calibration & Probing Blocks/motohawk_probe  nam='DeltaTPS'  show_more=on  name_source=Use Parameter  read_level=1  view_as=Number  enum_struct={'Disabled', 'Enabled'}  vector_style=Wide Row  use_help_units=off  help=''  units=''  use_header_enum=off  row_header_enum={}  col_header_enum={}  use_precision=off  precision=''  gain=1  offset=0  exp=1  use_mototune_group=on  mototune_group=motohawk_vardec_path(gcb)
  motohawk_probe3 : MotoHawk_lib/Calibration & Probing Blocks/motohawk_probe  nam='TransFuel_MAPFilt'  show_more=on  name_source=Use Parameter  read_level=1  view_as=Number  enum_struct={'Disabled', 'Enabled'}  vector_style=Wide Row  use_help_units=off  help=''  units=''  use_header_enum=off  row_header_enum={}  col_header_enum={}  use_precision=off  precision=''  gain=1  offset=0  exp=1  use_mototune_group=on  mototune_group=motohawk_vardec_path(gcb)
  motohawk_probe4 : MotoHawk_lib/Calibration & Probing Blocks/motohawk_probe  nam='TransFuel_TPSFilt'  show_more=on  name_source=Use Parameter  read_level=1  view_as=Number  enum_struct={'Disabled', 'Enabled'}  vector_style=Wide Row  use_help_units=off  help=''  units=''  use_header_enum=off  row_header_enum={}  col_header_enum={}  use_precision=off  precision=''  gain=1  offset=0  exp=1  use_mototune_group=on  mototune_group=motohawk_vardec_path(gcb)
  DeltaTPSMult : Outport  OutputWhenDisabled=reset  InitialOutput=1
  wires:
  Product1/1 -> DeltaTPSMult/1
  motohawk_prelookup/1 -> motohawk_interpolation_2d2/1, motohawk_interpolation_2d1/1
  motohawk_prelookup1/1 -> motohawk_interpolation_2d2/2
  MAF/1 -> motohawk_prelookup/1
  TPS/1 -> Sum/1, First Order Low Pass (Tunable)/1
  Sum/1 -> motohawk_prelookup1/1, motohawk_probe2/1
  First Order Low Pass (Tunable)/1 -> Sum/2, motohawk_probe4/1
  ECT Transient Fueling/1(Mult) -> Product1/2
  ECTIdx/1 -> ECT Transient Fueling/1(ECTIdx)
  motohawk_interpolation_2d2/1 -> Product1/1, CompareTo1/1
  motohawk_prelookup3/1 -> motohawk_interpolation_2d1/2
  MAPAngle/1 -> Sum1/1, First Order Low Pass (Tunable)1/1
  Sum1/1 -> motohawk_prelookup3/1, motohawk_probe1/1
  First Order Low Pass (Tunable)1/1 -> Sum1/2, motohawk_probe3/1
  motohawk_interpolation_2d1/1 -> Product1/3, CompareTo2/1
  OXY Transient Fueling/1(Mult) -> Product1/4
  OxyIdx/1 -> OXY Transient Fueling/1(OXYIdx)
  Logical Operator/1 -> ECT Transient Fueling/Enable, OXY Transient Fueling/Enable
  CompareTo1/1 -> Logical Operator/2
  CompareTo2/1 -> Logical Operator/1

== system BaseEngineController_LS_112/Foreground/Control/Controller/Run/Fuel System Manager/O2 Fuel Adapt/Adapt FuelFlowComp Map Bank A ==
  AdaptError : Inport
  Adapt : Inport  Port=2
  Enable : EnablePort
  Relational Operator1 : RelationalOperator  Operator=<=  OutDataTypeStr=boolean
  Relational Operator2 : RelationalOperator  OutDataTypeStr=boolean
  motohawk_adapt_table : MotoHawk_lib/Lookup Tables/motohawk_adapt_table  nam='FuelFlowCompAdapt_BankAMap'  typ=double  mode=Adapt only near a point  show_adapted=off
  motohawk_calibration1 : MotoHawk_lib/Calibration & Probing Blocks/motohawk_calibration  nam='FuelFlowCompMinValue_BankA'  val=0.5  storage=Calibration  show_more=on  name_source=Use Parameter  data_type=Inherit from 'Default Value'  read_level=1  write_level=1  ovr_cals=on  view_as=Number  enum_struct={'Disabled', 'Enabled'}  vector_style=Wide Row  use_help_units=on  help='Minimum value that can be adapted into the FuelFlowCompMap'  units='mult'  use_header_enum=off  row_header_enum={}  col_header_enum={}  use_min_max=on  min_val=0  max_val=2  use_precision=off  precision=''  gain=1  offset=0  exp=1  use_mototune_group=on  mototune_group=motohawk_vardec_path(gcb)
  motohawk_calibration2 : MotoHawk_lib/Calibration & Probing Blocks/motohawk_calibration  nam='FuelFlowCompMaxValue_BankA'  val=1.5  storage=Calibration  show_more=on  name_source=Use Parameter  data_type=Inherit from 'Default Value'  read_level=1  write_level=1  ovr_cals=on  view_as=Number  enum_struct={'Disabled', 'Enabled'}  vector_style=Wide Row  use_help_units=on  help='Maximum value that can be adapted into the FuelFlowCompMap'  units='mult'  use_header_enum=off  row_header_enum={}  col_header_enum={}  use_min_max=on  min_val=0  max_val=2  use_precision=off  precision=''  gain=1  offset=0  exp=1  use_mototune_group=on  mototune_group=motohawk_vardec_path(gcb)
  motohawk_fault_def : MotoHawk_lib/Fault Management Blocks/motohawk_fault_def  nam='FuelAdaptRangeHi_BankA'  mode=Enabled  id=[]  x=25  y=50  input_suspected=on  indeterminate=off  increment_xy=on  downsample_count=1  ovr_cals=on  ovr_actions=on  show_actions=off  action1_name=''  action1_cond=(None)  action2_name=''  action2_cond=(None)  action3_name=''  action3_cond=(None)  action4_name=''  action4_cond=(None)
  motohawk_fault_def1 : MotoHawk_lib/Fault Management Blocks/motohawk_fault_def  nam='FuelAdaptRangeLow_BankA'  mode=Enabled  id=[]  x=25  y=50  input_suspected=on  indeterminate=off  increment_xy=on  downsample_count=1  ovr_cals=on  ovr_actions=on  show_actions=off  action1_name=''  action1_cond=(None)  action2_name=''  action2_cond=(None)  action3_name=''  action3_cond=(None)  action4_name=''  action4_cond=(None)
  wires:
  Adapt/1 -> Relational Operator2/1, Relational Operator1/1
  Relational Operator1/1 -> motohawk_fault_def1/1
  Relational Operator2/1 -> motohawk_fault_def/1
  motohawk_calibration1/1 -> motohawk_adapt_table/2, Relational Operator1/2  "RichEquivRatioTargetDelta"
  AdaptError/1 -> motohawk_adapt_table/1  "RichEquivRatioTargetDelta"
  motohawk_calibration2/1 -> motohawk_adapt_table/3, Relational Operator2/2  "RichEquivRatioTargetDelta"

== system BaseEngineController_LS_112/Foreground/Control/Controller/Run/Fuel System Manager/O2 Fuel Adapt/Adapt FuelFlowComp Map Bank B ==
  AdaptError : Inport
  Adapt : Inport  Port=2
  Enable : EnablePort
  Relational Operator1 : RelationalOperator  Operator=<=  OutDataTypeStr=boolean
  Relational Operator2 : RelationalOperator  OutDataTypeStr=boolean
  motohawk_adapt_table : MotoHawk_lib/Lookup Tables/motohawk_adapt_table  nam='FuelFlowCompAdapt_BankBMap'  typ=double  mode=Adapt only near a point  show_adapted=off
  motohawk_calibration1 : MotoHawk_lib/Calibration & Probing Blocks/motohawk_calibration  nam='FuelFlowCompMinValue'  val=0.5  storage=Calibration  show_more=on  name_source=Use Parameter  data_type=Inherit from 'Default Value'  read_level=1  write_level=1  ovr_cals=on  view_as=Number  enum_struct={'Disabled', 'Enabled'}  vector_style=Wide Row  use_help_units=on  help='Minimum value that can be adapted into the FuelFlowCompMap'  units='mult'  use_header_enum=off  row_header_enum={}  col_header_enum={}  use_min_max=on  min_val=0  max_val=2  use_precision=off  precision=''  gain=1  offset=0  exp=1  use_mototune_group=on  mototune_group=motohawk_vardec_path(gcb)
  motohawk_calibration2 : MotoHawk_lib/Calibration & Probing Blocks/motohawk_calibration  nam='FuelFlowCompMaxValue'  val=1.5  storage=Calibration  show_more=on  name_source=Use Parameter  data_type=Inherit from 'Default Value'  read_level=1  write_level=1  ovr_cals=on  view_as=Number  enum_struct={'Disabled', 'Enabled'}  vector_style=Wide Row  use_help_units=on  help='Maximum value that can be adapted into the FuelFlowCompMap'  units='mult'  use_header_enum=off  row_header_enum={}  col_header_enum={}  use_min_max=on  min_val=0  max_val=2  use_precision=off  precision=''  gain=1  offset=0  exp=1  use_mototune_group=on  mototune_group=motohawk_vardec_path(gcb)
  motohawk_fault_def : MotoHawk_lib/Fault Management Blocks/motohawk_fault_def  nam='FuelAdaptRangeHi_BankB'  mode=Enabled  id=[]  x=25  y=50  input_suspected=on  indeterminate=off  increment_xy=on  downsample_count=1  ovr_cals=on  ovr_actions=on  show_actions=off  action1_name=''  action1_cond=(None)  action2_name=''  action2_cond=(None)  action3_name=''  action3_cond=(None)  action4_name=''  action4_cond=(None)
  motohawk_fault_def1 : MotoHawk_lib/Fault Management Blocks/motohawk_fault_def  nam='FuelAdaptRangeLow_BankB'  mode=Enabled  id=[]  x=25  y=50  input_suspected=on  indeterminate=off  increment_xy=on  downsample_count=1  ovr_cals=on  ovr_actions=on  show_actions=off  action1_name=''  action1_cond=(None)  action2_name=''  action2_cond=(None)  action3_name=''  action3_cond=(None)  action4_name=''  action4_cond=(None)
  wires:
  Adapt/1 -> Relational Operator2/1, Relational Operator1/1
  Relational Operator1/1 -> motohawk_fault_def1/1
  Relational Operator2/1 -> motohawk_fault_def/1
  motohawk_calibration1/1 -> motohawk_adapt_table/2, Relational Operator1/2  "RichEquivRatioTargetDelta"
  AdaptError/1 -> motohawk_adapt_table/1  "RichEquivRatioTargetDelta"
  motohawk_calibration2/1 -> motohawk_adapt_table/3, Relational Operator2/2  "RichEquivRatioTargetDelta"

== system BaseEngineController_LS_112/Foreground/Control/Controller/Run/Fuel System Manager/O2 Fuel Adapt/O2 Control Enable Delay ==
  State_In : Inport
  Relational Operator : RelationalOperator  Operator=>  InputSameDT=on
  Time Since Enabled (With Input)1 : motohawk_control_primitives_lib/Time Since Enabled (With Input)1  SystemSampleTime=-1  nam='LiqDelayTime'  samp_time=.005  init=0  upperlim=16000
  motohawk_calibration1 : MotoHawk_lib/Calibration & Probing Blocks/motohawk_calibration  nam='O2CtrlAdaptDelayTime'  val=5  storage=Calibration  show_more=on  name_source=Use Parameter  data_type=Inherit from 'Default Value'  read_level=1  write_level=1  ovr_cals=on  view_as=Number  enum_struct={'Disabled', 'Enabled'}  vector_style=Wide Row  use_help_units=on  help='O2 Control must be enabled for this amount of time before fuel adaption is enabled'  units='s'  use_header_enum=off  row_header_enum={}  col_header_enum={}  use_min_max=off  min_val=0  max_val=inf  use_precision=off  precision=''  gain=1  offset=0  exp=1  use_mototune_group=on  mototune_group=motohawk_vardec_path(gcb)
  State_Out : Outport
  wires:
  State_In/1 -> Time Since Enabled (With Input)1/1
  motohawk_calibration1/1 -> Relational Operator/2
  Time Since Enabled (With Input)1/1 -> Relational Operator/1
  Relational Operator/1 -> State_Out/1

== system BaseEngineController_LS_112/Foreground/Control/Controller/Run/Fuel System Manager/O2 Fuel Adapt/Saturation (Tunable) ==
  note: Calibratable wrapper around the Saturation block
  In : Inport
  Saturation : motohawk_control_primitives_lib/Saturation  SystemSampleTime=-1
  motohawk_calibration : MotoHawk_lib/Calibration & Probing Blocks/motohawk_calibration  nam=[prefix 'LwrLim']  val=LwrLim  storage=Calibration  show_more=on  name_source=Use Parameter  data_type=Inherit via back propagation  read_level=1  write_level=1  ovr_cals=on  view_as=Number  enum_struct={'Disabled', 'Enabled'}  vector_style=Wide Row  use_help_units=off  help='Lower Limit Value'  units=units  use_header_enum=off  row_header_enum={}  col_header_enum={}  use_min_max=on  min_val=-inf  max_val=inf  use_precision=on  precision='1.4'  gain=1  offset=0  exp=1  use_mototune_group=on  mototune_group=motohawk_vardec_path(gcb)
  motohawk_calibration1 : MotoHawk_lib/Calibration & Probing Blocks/motohawk_calibration  nam=[prefix 'UprLim']  val=UprLim  storage=Calibration  show_more=on  name_source=Use Parameter  data_type=Inherit via back propagation  read_level=1  write_level=1  ovr_cals=on  view_as=Number  enum_struct={'Disabled', 'Enabled'}  vector_style=Wide Row  use_help_units=off  help='Upper Limit Value'  units=units  use_header_enum=off  row_header_enum={}  col_header_enum={}  use_min_max=on  min_val=-inf  max_val=inf  use_precision=on  precision='1.4'  gain=1  offset=0  exp=1  use_mototune_group=on  mototune_group=motohawk_vardec_path(gcb)
  Out : Outport
  wires:
  motohawk_calibration1/1 -> Saturation/3
  In/1 -> Saturation/1
  motohawk_calibration/1 -> Saturation/2
  Saturation/1 -> Out/1
